simulink library "ESTS_UOD_FacUnderSteer"  (R2022a)
settings: Solver=VariableStepAuto  StartTime=0.0  StopTime=10.0  RelTol=1e-3
undefined symbols (not defined in the file or in its folder): ESTS_UOD_c_TiSample_s, ESTS_UOD_p_AgrVSideSlipReDifLatRefLimUS_degps, ESTS_UOD_p_TiTrans_s, ESTS_UOD_p_YawRateDifLatRefLimUS_degps
libraries: VUT_lib x2, simulink x1
settings Model: Creator=blatak  LastModifiedBy=blatak

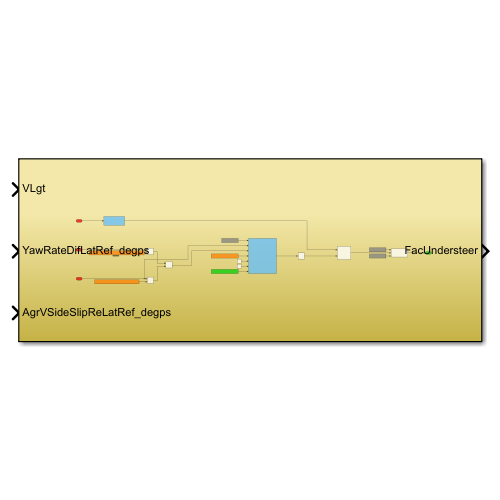
[thumbnail: Simulink's stored preview of the top-level diagram]
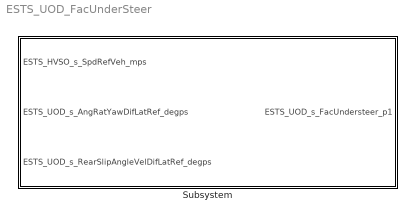
== system ESTS_UOD_FacUnderSteer ==
  Subsystem : Subsystem

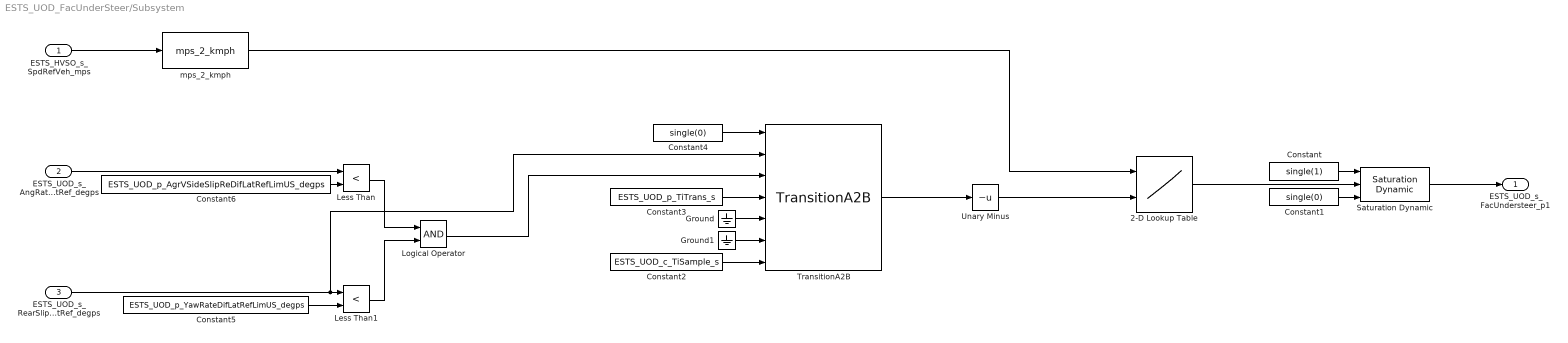
== system ESTS_UOD_FacUnderSteer/Subsystem ==
  ESTS_HVSO_s_SpdRefVeh_mps : Inport
  ESTS_UOD_s_AngRatYawDifLatRef_degps : Inport  Port=2
  ESTS_UOD_s_RearSlipAngleVelDifLatRef_degps : Inport  Port=3
  2-D Lookup Table : Lookup_n-D  BreakpointsForDimension1=[1:3]  BreakpointsForDimension2=[1:3]  InternalRulePriority=Speed  RndMeth=Simplest
      settings: InputPortMap=u0,u1
  Constant : Constant  Value=single(1)
  Constant1 : Constant  Value=single(0)
  Constant2 : Constant  Value=ESTS_UOD_c_TiSample_s
  Constant3 : Constant  Value=ESTS_UOD_p_TiTrans_s
  Constant4 : Constant  Value=single(0)
  Constant5 : Constant  Value=ESTS_UOD_p_YawRateDifLatRefLimUS_degps
  Constant6 : Constant  Value=ESTS_UOD_p_AgrVSideSlipReDifLatRefLimUS_degps
  Ground : Ground
  Ground1 : Ground
  Less Than : RelationalOperator  Operator=<  OutDataTypeStr=boolean  RndMeth=Simplest  InputSameDT=off
  Less Than1 : RelationalOperator  Operator=<  OutDataTypeStr=boolean  RndMeth=Simplest  InputSameDT=off
  Logical Operator : Logic  AllPortsSameDT=off  OutDataTypeStr=boolean
  Saturation Dynamic : simulink/Discontinuities/Saturation Dynamic  OutMin=[]  OutMax=[]  OutDataTypeStr=Inherit: Same as second input  OutDataType=fixdt(1, 16)  OutScaling=2^-10  DoSatur=off
  TransitionA2B : VUT_lib/TransitionA2B  SystemSampleTime=-1  VariantActivationTime=update diagram  Latency=0  AutoFrameSizeCalculation=off
  Unary Minus : UnaryMinus
  mps_2_kmph : VUT_lib/mps_2_kmph  SystemSampleTime=-1  VariantActivationTime=update diagram  Latency=0  AutoFrameSizeCalculation=off
  ESTS_UOD_s_FacUndersteer_p1 : Outport
  wires:
  Unary Minus/1 -> 2-D Lookup Table/2
  Ground/1 -> TransitionA2B/5
  2-D Lookup Table/1 -> Saturation Dynamic/2
  Constant4/1 -> TransitionA2B/1
  ESTS_UOD_s_RearSlipAngleVelDifLatRef_degps/1 -> TransitionA2B/2, Less Than1/1
  Constant1/1 -> Saturation Dynamic/3
  Constant/1 -> Saturation Dynamic/1
  Saturation Dynamic/1 -> ESTS_UOD_s_FacUndersteer_p1/1
  Less Than1/1 -> Logical Operator/2
  Logical Operator/1 -> TransitionA2B/3
  Constant2/1 -> TransitionA2B/7
  Constant5/1 -> Less Than1/2
  TransitionA2B/1 -> Unary Minus/1
  ESTS_UOD_s_AngRatYawDifLatRef_degps/1 -> Less Than/1
  Constant6/1 -> Less Than/2
  Less Than/1 -> Logical Operator/1
  Constant3/1 -> TransitionA2B/4
  ESTS_HVSO_s_SpdRefVeh_mps/1 -> mps_2_kmph/1
  Ground1/1 -> TransitionA2B/6
  mps_2_kmph/1 -> 2-D Lookup Table/1
